simulink model "Fall_Detection"  (R2023a)
settings: Solver=FixedStepAuto  StartTime=0.0  StopTime=inf  RelTol=1e-3
libraries: androidsensorlib x4, androiduilib x3
settings Model: Creator=Rakesh  LastModifiedBy=Rakesh
settings OptimizationCC: EnhancedBackFolding=on  PassReuseOutputArgsAs=Individual arguments  ZeroExternalMemoryAtStartup=off  ZeroInternalMemoryAtStartup=off  MaxStackSize=64  OptimizeBlockOrder=speed  DifferentSizesBufferReuse=on  OptimizationCustomize=off  EfficientTunableParamExpr=on
settings DebuggingCC: ParameterTunabilityLossMsg=error
settings HardwareCC: ProdBitPerPointer=32  ProdBitPerSizeT=32  ProdBitPerPtrDiffT=32  ProdLargestAtomicInteger=Long  ProdLargestAtomicFloat=Double  ProdWordSize=32  ProdHWDeviceType=ARM Compatible->ARM Cortex  UseEmbeddedCoderFeatures=off  UseSimulinkCoderFeatures=off
settings SFSimCC: MATLABDynamicMemAlloc=off
settings RTWCC: Description=Embedded Coder  SystemTargetFile=ert.tlc  HardwareBoard=Android Device  TLCOptions="-aInlineSetEventsForThisBaseRateFcn=TLC_FALSE -aSuppressMultiTaskScheduler=TLC_FALSE  -aRateBasedStepFcn=0"  TemplateMakefile=ert_default_tmf  RTWVerbose=off  Toolchain=Android SDK/NDK Tools
settings CodeAppCC: ForceParamTrailComments=on  IgnoreCustomStorageClasses=off  OperatorAnnotations=on  SimulinkDataObjDesc=on  SFDataObjDesc=on  InsertBlockDesc=on
settings ERTTargetCC: SupportNonInlinedSFcns=on

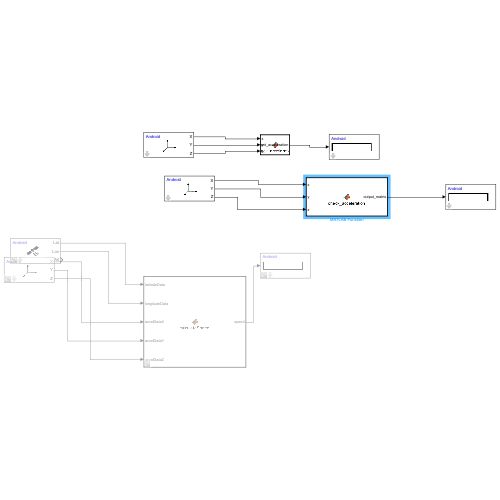
[thumbnail: Simulink's stored preview of the top-level diagram]
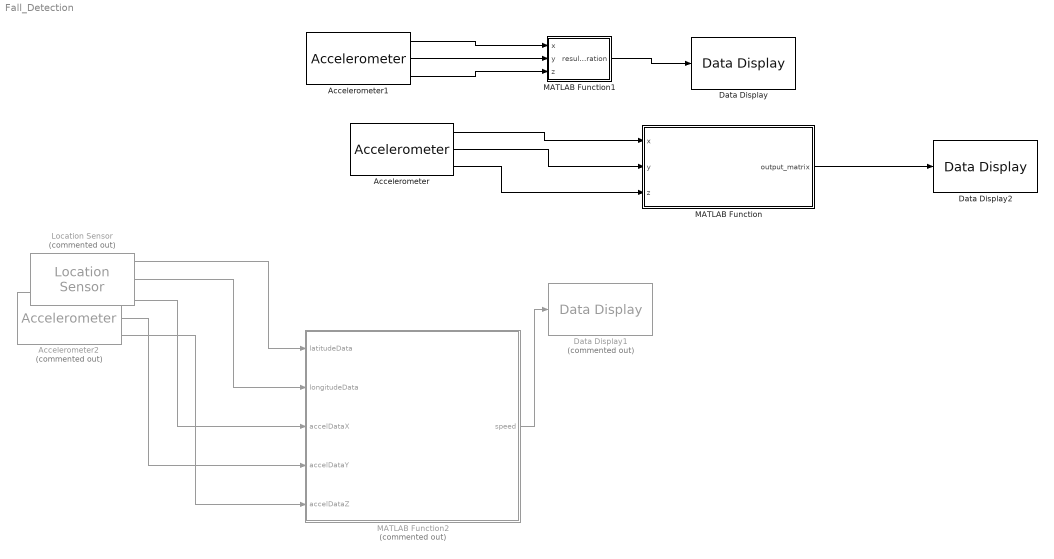
== system Fall_Detection ==
  Accelerometer : androidsensorlib/Accelerometer  OutputVector=off  SampleTime=0.1  BlockPlatform=Android
  Accelerometer1 : androidsensorlib/Accelerometer  OutputVector=off  SampleTime=0.1  BlockPlatform=Android
  Accelerometer2 : androidsensorlib/Accelerometer  Commented=on  OutputVector=off  SampleTime=0.1  BlockPlatform=Android
  Data Display : androiduilib/Data Display  DataDisplayId=Fall_Detection/Data_Display  Format=Float  Precision=6  SimulateUsing=Code generation  blockPlatform=Android
  Data Display1 : androiduilib/Data Display  Commented=on  DataDisplayId=Fall_Detection/Data_Display1  Format=Float  Precision=6  SimulateUsing=Code generation  blockPlatform=Android
  Data Display2 : androiduilib/Data Display  DataDisplayId=Fall_Detection/Data_Display2  Format=Float  Precision=6  SimulateUsing=Code generation  blockPlatform=Android
  Location Sensor : androidsensorlib/Location Sensor  Commented=on  OutputVector=off  SampleTime=0.1  BlockPlatform=Android
  MATLAB Function : MATLAB Function  TreatAsAtomicUnit=on
  MATLAB Function1 : MATLAB Function  TreatAsAtomicUnit=on
  MATLAB Function2 : MATLAB Function  Commented=on  TreatAsAtomicUnit=on
  wires:
  Accelerometer/1 -> MATLAB Function/1(x)
  Accelerometer/2 -> MATLAB Function/2(y)
  Accelerometer/3 -> MATLAB Function/3(z)
  Accelerometer1/1 -> MATLAB Function1/1(x)
  Accelerometer1/2 -> MATLAB Function1/2(y)
  Accelerometer1/3 -> MATLAB Function1/3(z)
  MATLAB Function1/1(resultant_acceleration) -> Data Display/1
  Location Sensor/1 -> MATLAB Function2/1(latitudeData)
  Location Sensor/2 -> MATLAB Function2/2(longitudeData)
  Accelerometer2/1 -> MATLAB Function2/3(accelDataX)
  Accelerometer2/2 -> MATLAB Function2/4(accelDataY)
  Accelerometer2/3 -> MATLAB Function2/5(accelDataZ)
  MATLAB Function2/1(speed) -> Data Display1/1
  MATLAB Function/1(output_matrix) -> Data Display2/1

== matlab function Fall_Detection/MATLAB Function1 ==
  data: x input; resultant_acceleration output; y input; z input
function resultant_acceleration = check_acceleration(x, y, z)   
    resultant_acceleration = sqrt(x^2 + y^2 + z^2);
end

== matlab function Fall_Detection/MATLAB Function ==
  data: x input; output_matrix output; y input; z input
function output_matrix  = check_acceleration(x, y, z)
    resultant_acceleration = sqrt(x^2 + y^2 + z^2);
    exceeds_threshold = resultant_acceleration > 10;
    if exceeds_threshold;
        %fs = 44100;  
        %duration = 1;  
        %frequency = 440;  
        %t = linspace(0, duration, fs*duration);  
        %waveform = sin(2*pi*frequency*t); 
        output_matrix=6;
        %output_matrix = [int16(waveform'), int16(waveform')];  
        %output_matrix = int16(ones(4410, 2));
    else
        %output_matrix = int16(zeros(4410, 2));
        output_matrix = 7;
    end
end

== matlab function Fall_Detection/MATLAB Function2 ==
  data: latitudeData input; speed output; longitudeData input; accelDataX input; accelDataY input; accelDataZ input
function speed = calculateSpeed(latitudeData, longitudeData, accelDataX, accelDataY, accelDataZ)
    % Initialize variables
    dt = 0.1; % Time step in seconds
    numSamples = length(latitudeData);
    speed = zeros(numSamples, 1);
    
    % Kalman filter parameters
    Q = 0.01; % Process noise covariance
    R = 0.1; % Measurement noise covariance
    x = 0; % Initial state estimate
    P = 1; % Initial error covariance
    
    % Iterate over the data
    for i = 2:numSamples
        % Prediction step
        x = x; % No change in speed prediction
        P = P + Q; % Update error covariance
        
        % Update step
        K = P / (P + R); % Kalman gain
        deltaLatitude = latitudeData(i) - latitudeData(i-1); % Change in latitude
        deltaLongitude = longitudeData(i) - longitudeData(i-1); % Change in longitude
        distance_gps = sqrt(deltaLatitude^2 + deltaLongitude^2); % Distance between consecutive GPS points
        
        accelMagnitude = sqrt(accelDataX(i)^2 + accelDataY(i)^2 + accelDataZ(i)^2); % Magnitude of accelerometer data
        
        % Estimate speed based on accelerometer data
        accel_speed = accelMagnitude * dt;
        
        % Combine GPS and accelerometer data for speed estimation
        speed(i) = (distance_gps / dt) + accel_speed;
        
        x = x + K * (speed(i) - x); % Update state estimate
        P = (1 - K) * P; % Update error covariance
    end
end
